simulink library "sun_sensor_lib"  (R2018b)
settings: Solver=VariableStepAuto  StartTime=0.0  StopTime=10.0  RelTol=1e-3
undefined symbols (not defined in the file): simParams
libraries: simulink x2, vrlib x1, aerolibutil x1, ss_vec_2_angles x1
settings Model: Creator=colem  LastModifiedBy=taylorreynolds

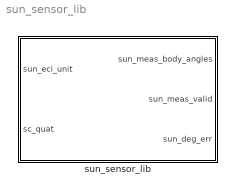
== system sun_sensor_lib ==
  "sun_sensor_lib " : Subsystem

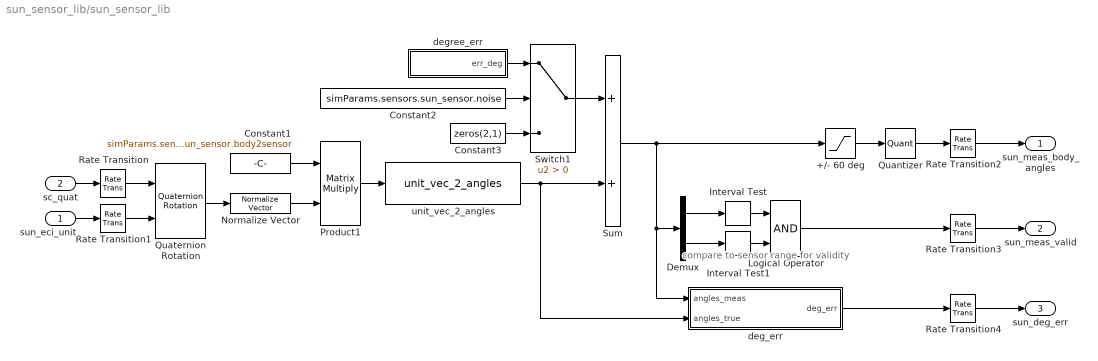
== system sun_sensor_lib/sun_sensor_lib  ==
  note: compare to sensor range for validity
  sun_eci_unit : Inport
  sc_quat : Inport  Port=2
  +/- 60 deg : Saturate  UpperLimit=simParams.sensors.sun_sensor.range_deg  LowerLimit=-simParams.sensors.sun_sensor.range_deg
  Constant1 : Constant  Value=simParams.sensors.sun_sensor.body2sensor
  Constant2 : Constant  Value=simParams.sensors.sun_sensor.noise
  Constant3 : Constant  Value=zeros(2,1)
  Demux : Demux  Outputs=2
  Interval Test : simulink/Logic and Bit Operations/Interval Test  IntervalClosedRight=on  uplimit=simParams.sensors.sun_sensor.range_deg  IntervalClosedLeft=on  lowlimit=-simParams.sensors.sun_sensor.range_deg  OutDataTypeStr=boolean
  Interval Test1 : simulink/Logic and Bit Operations/Interval Test  IntervalClosedRight=on  uplimit=simParams.sensors.sun_sensor.range_deg  IntervalClosedLeft=on  lowlimit=-simParams.sensors.sun_sensor.range_deg  OutDataTypeStr=boolean
  Logical Operator : Logic  AllPortsSameDT=off  OutDataTypeStr=boolean
  Normalize Vector : vrlib/Utilities/Normalize Vector  maxzero=0
      settings: SourceProductName=Simulink 3D Animation  SourceProductBaseCode=VR
  Product1 : Product  Multiplication=Matrix(*)  RndMeth=Zero
  Quantizer : Quantizer  QuantizationInterval=simParams.sensors.sun_sensor.resolution
  Quaternion Rotation : aerolibutil/Quaternion Rotation
  Rate Transition : RateTransition  InitialCondition=simParams.initialConditions.q_eci2body  OutPortSampleTime=simParams.sensors.sun_sensor.sample_time_s
  Rate Transition1 : RateTransition  OutPortSampleTime=simParams.sensors.sun_sensor.sample_time_s
  Rate Transition2 : RateTransition
  Rate Transition3 : RateTransition
  Rate Transition4 : RateTransition
  Sum : Sum
  Switch1 : Switch  Criteria=u2 > Threshold
  deg_err : Subsystem
  degree_err : Subsystem
  unit_vec_2_angles : ss_vec_2_angles/unit_vec_2_angles  SystemSampleTime=-1
  sun_meas_body_angles : Outport
  sun_meas_valid : Outport  Port=2
  sun_deg_err : Outport  Port=3
  wires:
  sc_quat/1 -> Rate Transition/1
  Constant2/1 -> Switch1/2
  Constant3/1 -> Switch1/3
  Switch1/1 -> Sum/1
  sun_eci_unit/1 -> Rate Transition1/1
  deg_err/1(deg_err) -> Rate Transition4/1
  degree_err/1("err_deg ") -> Switch1/1
  Quaternion Rotation/1 -> Normalize Vector/1
  Quantizer/1 -> Rate Transition2/1
  Normalize Vector/1 -> Product1/2
  Demux/1 -> Interval Test/1
  Interval Test/1 -> Logical Operator/1
  Interval Test1/1 -> Logical Operator/2
  +/- 60 deg/1 -> Quantizer/1
  Constant1/1 -> Product1/1
  Product1/1 -> unit_vec_2_angles/1
  unit_vec_2_angles/1 -> Sum/2, deg_err/2(angles_true)
  Sum/1 -> +/- 60 deg/1, deg_err/1(angles_meas), Demux/1
  Demux/2 -> Interval Test1/1
  Logical Operator/1 -> Rate Transition3/1
  Rate Transition/1 -> Quaternion Rotation/1
  Rate Transition1/1 -> Quaternion Rotation/2
  Rate Transition2/1 -> sun_meas_body_angles/1
  Rate Transition3/1 -> sun_meas_valid/1
  Rate Transition4/1 -> sun_deg_err/1

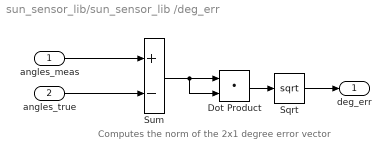
== system sun_sensor_lib/sun_sensor_lib /deg_err ==
  note: Computes the norm of the 2x1 degree error vector
  angles_meas : Inport
  angles_true : Inport  Port=2
  Dot Product : DotProduct  InputSameDT=on  OutDataTypeStr=Inherit: Inherit via internal rule
  Sqrt : Sqrt  SaturateOnIntegerOverflow=on
  Sum : Sum  Inputs=+-
  deg_err : Outport
  wires:
  angles_meas/1 -> Sum/1
  angles_true/1 -> Sum/2
  Sum/1 -> Dot Product/2, Dot Product/1
  Dot Product/1 -> Sqrt/1
  Sqrt/1 -> deg_err/1

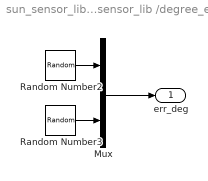
== system sun_sensor_lib/sun_sensor_lib /degree_err ==
  Mux : Mux  Inputs=2
  Random Number2 : RandomNumber  Variance=simParams.sensors.sun_sensor.deg_var  Seed=simParams.sensors.sun_sensor.seed(1)  SampleTime=simParams.sensors.sun_sensor.sample_time_s
  Random Number3 : RandomNumber  Variance=simParams.sensors.sun_sensor.deg_var  Seed=simParams.sensors.sun_sensor.seed(2)  SampleTime=simParams.sensors.sun_sensor.sample_time_s
  "err_deg " : Outport
  wires:
  Random Number2/1 -> Mux/1
  Random Number3/1 -> Mux/2
  Mux/1 -> "err_deg "/1
